simulink model "final_3_simu_20241216"  (R2021a)
settings: Solver=VariableStepAuto  StartTime=0.0  StopTime=10.0  RelTol=1e-3
libraries: cstblocks x1
settings Model: Creator=frand  LastModifiedBy=frand

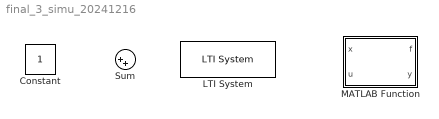
== system final_3_simu_20241216 ==
  Constant : Constant
  LTI System : cstblocks/LTI System  sys=C_dig  IC=[]
  MATLAB Function : MATLAB Function  TreatAsAtomicUnit=on
  Sum : Sum  Inputs=|++

== matlab function final_3_simu_20241216/MATLAB Function ==
  data: x input; f output; u input; y output
function [f,y] = fcn(x,u)

p = 0.02;

f1 = 

f = [f1;f2;f3];

y = u;
